simulink model "SimulinkModel_PID_SecondTest"  (R2020a)
settings: Solver=ode14x  StartTime=0.0  StopTime=SimTime  FixedStep=solverTimeStep  RelTol=1e-3
InitFcn:
  | StartupScript
values from neighbouring files (symbols this model uses):
  B = B*GearRatio^2    (= 0.0676821220781)    [StartupScript.m]
  CF = 1000.0    (= 1000)    [StartupScript.m]
  GearRatio = 111.0    (= 111)    [StartupScript.m]
  J = J*GearRatio^2    (= 0.13885767)    [StartupScript.m]
  K = 1.0    (= 1)    [StartupScript.m]
  Kd = 0.05    [StartupScript.m]
  Ki = 0.00    (= 0)    [StartupScript.m]
  Km = 23.4*1e-3    (= 0.0234)    [StartupScript.m]
  Kp = 2.8    [StartupScript.m]
  L = 0.0774e-3    (= 7.74e-05)    [StartupScript.m]
  R = 0.212    [StartupScript.m]
  r2d = 180/pi    (= 57.2957795131)    [StartupScript.m]
  sensorGain = 150.0    (= 150)    [StartupScript.m]
libraries: cstblocks x1
settings Model: Creator=nisch  LastModifiedBy=nisch

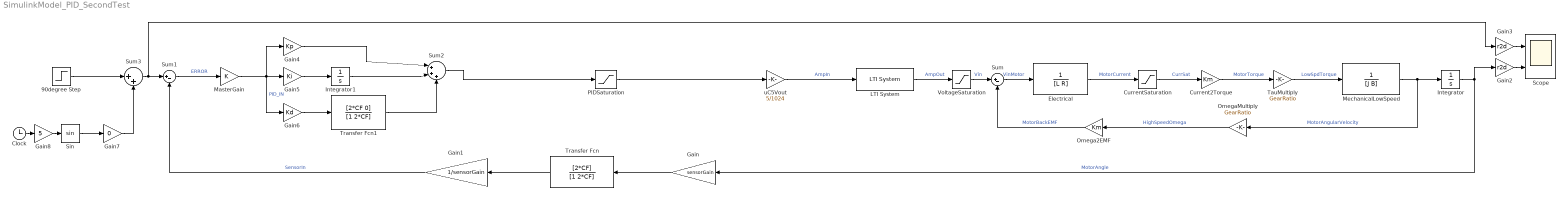
== system SimulinkModel_PID_SecondTest ==
  90degree Step : Step  Time=0  After=pi/2  SampleTime=0
  Clock : Clock
  Current2Torque : Gain  Gain=Km
  CurrentSaturation : Saturate  UpperLimit=10  LowerLimit=-10
  Electrical : TransferFcn  Denominator=[L R]
  Gain : Gain  Gain=sensorGain
  Gain1 : Gain  Gain=1/sensorGain
  Gain2 : Gain  Gain=r2d
  Gain3 : Gain  Gain=r2d
  Gain4 : Gain  Gain=Kp
  Gain5 : Gain  Gain=Ki
  Gain6 : Gain  Gain=Kd
  Gain7 : Gain  Gain=0
  Gain8 : Gain  Gain=5
  Integrator : Integrator
  Integrator1 : Integrator
  LTI System : cstblocks/LTI System  sys=VoltageAmplifier  IC=[]
  MasterGain : Gain  Gain=K
  MechanicalLowSpeed : TransferFcn  Denominator=[J B]
  Omega2EMF : Gain  Gain=Km
  OmegaMultiply : Gain  Gain=GearRatio
  PIDSaturation : Saturate  UpperLimit=1024  LowerLimit=-1024
  Scope : Scope  NumInputPorts=2
  Sin : Trigonometry
  Sum : Sum  Inputs=|+-
  Sum1 : Sum  Inputs=|+-
  Sum2 : Sum  Inputs=|+++
  Sum3 : Sum  Inputs=|++
  TauMultiply : Gain  Gain=GearRatio
  Transfer Fcn : TransferFcn  Numerator=[2*CF]  Denominator=[1 2*CF]
  Transfer Fcn1 : TransferFcn  Numerator=[2*CF 0]  Denominator=[1 2*CF]
  VoltageSaturation : Saturate  UpperLimit=18  LowerLimit=-18
  uC5Vout : Gain  Gain=5/1024
  wires:
  Sum/1 -> Electrical/1  "VinMotor"
  Omega2EMF/1 -> Sum/2  "MotorBackEMF"
  MechanicalLowSpeed/1 -> Integrator/1, OmegaMultiply/1  "MotorAngularVelocity"
  Sum1/1 -> MasterGain/1  "ERROR"
  Integrator/1 -> Gain2/1, Gain/1  "MotorAngle"
  Gain/1 -> Transfer Fcn/1
  Transfer Fcn/1 -> Gain1/1
  Gain1/1 -> Sum1/2  "SensorIn"
  Gain2/1 -> Scope/2
  Gain3/1 -> Scope/1
  VoltageSaturation/1 -> Sum/1  "Vin"
  MasterGain/1 -> Gain6/1, Gain5/1, Gain4/1  "PID_IN"
  Gain5/1 -> Integrator1/1
  Gain6/1 -> Transfer Fcn1/1
  Sum2/1 -> PIDSaturation/1
  Gain4/1 -> Sum2/1
  Integrator1/1 -> Sum2/2
  Transfer Fcn1/1 -> Sum2/3
  Electrical/1 -> CurrentSaturation/1  "MotorCurrent"
  CurrentSaturation/1 -> Current2Torque/1  "CurrSat"
  Current2Torque/1 -> TauMultiply/1  "MotorTorque"
  TauMultiply/1 -> MechanicalLowSpeed/1  "LowSpdTorque"
  OmegaMultiply/1 -> Omega2EMF/1  "HighSpeedOmega"
  Sum3/1 -> Gain3/1, Sum1/1
  90degree Step/1 -> Sum3/1
  Sin/1 -> Gain7/1
  Gain7/1 -> Sum3/2
  Clock/1 -> Gain8/1
  Gain8/1 -> Sin/1
  LTI System/1 -> VoltageSaturation/1  "AmpOut"
  PIDSaturation/1 -> uC5Vout/1
  uC5Vout/1 -> LTI System/1  "AmpIn"
